simulink model "hvac_maborrelli_singapur_nzones_TCH2"  (R2021a)
settings: Solver=ode45  StartTime=0.0  StopTime=Inf  FixedStep=2  RelTol=1e-3  EnableMultiTasking=on
values from neighbouring files (symbols this model uses):
  beta = 0.15    [main_td3_nzones.m]
  ci = ci'    [localResetFcn.m]    (also in localResetFcnT.m)
  CO2_max = 1200*1e-6    (= 0.0012)    [main_td3_nzones.m]
  high = 25    [main_td3_nzones.m]    (also in reward.m)
  low = -10    [isDone.m]    (also in main_td3_nzones.m = 22; reward.m = 22)
  params = params1    [main_td3_nzones.m]
  paramsnz =     [values4z_tch.mat]
  scale = limit_act_low + limit_act_h    [main_td3_nzones.m]
  Ts = delta*Tr+(1-delta)*Toa + DT + DTH    [dynamics_hvac_maborrelli_singapur_1zone_tch.m]    (also in main_td3_nzones.m = 60)
  Ts2 = 900    [main.m]    (also in main_td3_nzones.m = 600)
undefined symbols (not defined in the file or in its folder): id, rl
libraries: simulink x6, dspmathops x5, rllib x1
settings Model: Creator=User  LastModifiedBy=Richi
settings SolverCC: AlgebraicLoopSolver=TrustRegion
settings DataIOCC: LimitDataPoints=on  SaveFormat=Array  SignalLoggingSaveFormat=ModelDataLogs
settings OptimizationCC: LifeSpan=inf
settings DebuggingCC: SolverPrmCheckMsg=warning  MultiTaskDSMMsg=warning  MultiTaskCondExecSysMsg=none  MultiTaskRateTransMsg=warning  StrictBusMsg=ErrorOnBusTreatedAsVector  SFUnexpectedBacktrackingDiag=warning  SFNoUnconditionalDefaultTransitionDiag=warning  SFExecutionAtInitializationDiag=none  SFMachineParentedDataDiag=warning  ArithmeticOperatorsInVariantConditions=warning
settings HardwareCC: ProdBitPerPointer=32  ProdBitPerSizeT=32  ProdBitPerPtrDiffT=32  ProdLargestAtomicFloat=None  ProdIntDivRoundTo=Undefined  ProdEndianess=Unspecified  ProdWordSize=32  ProdHWDeviceType=32-bit Generic
settings ModelReferenceCC: PropagateSignalLabelsOutOfModel=off
settings SFSimCC: SimUseLocalCustomCode=off  CustomCodeUndefinedFunction=UseInterfaceOnly
settings RTWCC: RTWUseLocalCustomCode=off
settings CodeAppCC: StateflowObjectComments=on
settings GRTTargetCC: TargetLangStandard=C89/C90 (ANSI)
settings ConfigComp: CovMetricSettings=dw  CovSaveCumulativeToWorkspaceVar=on  CovSaveSingleToWorkspaceVar=on  CovExternalEMLEnable=off

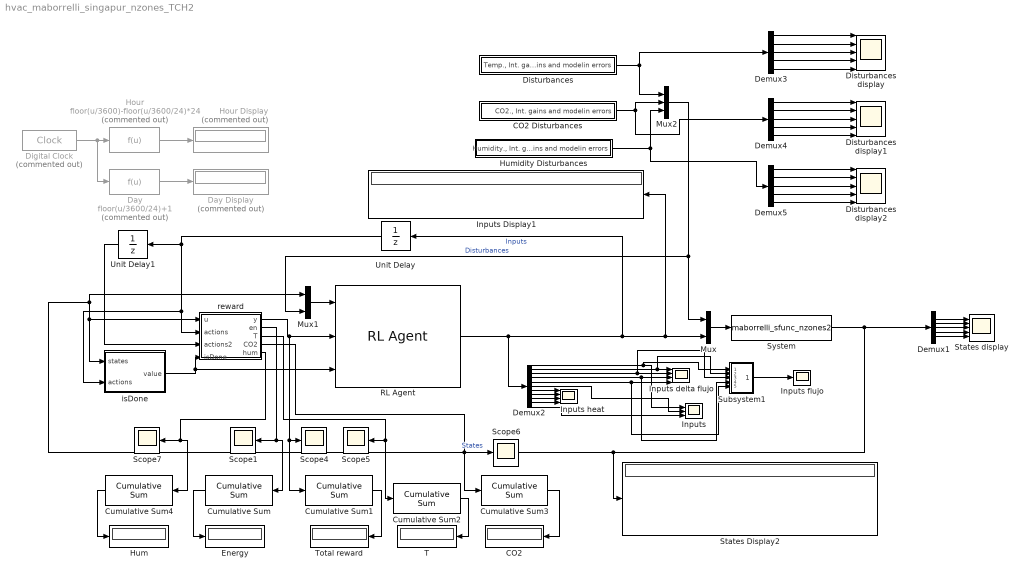
== system hvac_maborrelli_singapur_nzones_TCH2 ==
  CO2 : Display
  CO2 Disturbances : Subsystem  TreatAsAtomicUnit=on
  Cumulative Sum{,1..4} (5 alike) : dspmathops/Cumulative Sum  dim=Channels (running sum)  InputProcessing=Columns as channels (frame based)  reset_popup=None  roundingMode=Floor  overflowMode=off  outputDataTypeStr=Inherit: Same as accumulator  outputMin=[]  outputMax=[]  outputLastDataTypeStr=Inherit: Same as accumulator
  Day : Fcn  Commented=on  Expr=floor(u/3600/24)+1  SampleTime=1800
  Day Display : Display  Commented=on
  Demux{1,3..5} (4 alike) : Demux  Outputs=5
  Demux2 : Demux  Outputs=11
  Digital Clock : DigitalClock  Commented=on  SampleTime=60
  Disturbances : Subsystem  TreatAsAtomicUnit=on
  Disturbances display : Scope  NumInputPorts=5
  Disturbances display1 : Scope  NumInputPorts=5
  Disturbances display2 : Scope  NumInputPorts=5
  Energy : Display
  Hour : Fcn  Commented=on  Expr=floor(u/3600)-floor(u/3600/24)*24  SampleTime=1800
  Hour Display : Display  Commented=on
  Hum : Display
  Humidity Disturbances : Subsystem  TreatAsAtomicUnit=on
  "Inputs " : Scope  NumInputPorts=3
  Inputs Display1 : Display
  Inputs delta flujo : Scope  NumInputPorts=4
  Inputs flujo : Scope
  Inputs heat : Scope  NumInputPorts=4
  Mux : Mux  Inputs=2
  Mux1 : Mux  Inputs=2
  Mux2 : Mux  Inputs=3
  RL Agent : rllib/RL Agent  Agent=rl.util.PolicyInstance.get('hvac_maborrelli_singapur_nzones_with_MPC_v3_manualdist_3/RL Agent')  ExternalActionAsInput=off  ProvideCumRwd=off  TreatAsDirectFeedthrough=on
  Scope{1,4..7} (5 alike) : Scope
  States Display2 : Display
  States display : Scope  NumInputPorts=5
  Subsystem1 : Subsystem
  System : S-Function  FunctionName=maborrelli_sfunc_nzones2  Parameters=ci,paramsnz,Ts  SFunctionDeploymentMode=off  EnableBusSupport=off
  T : Display
  Total reward : Display
  Unit Delay : UnitDelay  SampleTime=Ts2  HasFrameUpgradeWarning=on
  Unit Delay1 : UnitDelay  SampleTime=Ts2  HasFrameUpgradeWarning=on
  isDone : MATLAB Function  TreatAsAtomicUnit=on
  reward : MATLAB Function  TreatAsAtomicUnit=on
  wires:
  Mux/1 -> System/1
  System/1 -> Demux1/1, States Display2/1, Mux1/1, isDone/1(states), reward/1(u)  "States"
  RL Agent/1 -> Unit Delay/1, Mux/2, Inputs Display1/1, Demux2/1  "Inputs"
  Hour/1 -> Hour Display/1
  Digital Clock/1 -> Day/1, Hour/1
  Day/1 -> Day Display/1
  Demux1/1 -> States display/1
  Demux1/2 -> States display/2
  Demux1/3 -> States display/3
  Demux1/4 -> States display/4
  isDone/1(value) -> reward/4(isDone), RL Agent/3
  Mux1/1 -> RL Agent/1
  Unit Delay/1 -> Unit Delay1/1, isDone/2(actions), reward/2(actions)
  Disturbances/1("Temp., Int. gains and modelin errors") -> Mux2/1, Demux3/1
  CO2 Disturbances/1("CO2., Int. gains and modelin errors") -> Mux2/2, Demux4/1
  Humidity Disturbances/1("Humidity., Int. gains and modelin errors") -> Demux5/1, Mux2/3
  Mux2/1 -> Mux1/2, Mux/1  "Disturbances"
  Demux3/1 -> Disturbances display/1
  Cumulative Sum4/1 -> Hum/1
  reward/4(CO2) -> Cumulative Sum3/1, Scope6/1
  Cumulative Sum/1 -> Energy/1
  Cumulative Sum2/1 -> T/1
  reward/5(hum) -> Cumulative Sum4/1, Scope7/1
  Cumulative Sum3/1 -> CO2/1
  reward/1(y) -> Cumulative Sum1/1, Scope4/1, RL Agent/2
  reward/3(T) -> Cumulative Sum2/1, Scope5/1
  Cumulative Sum1/1 -> Total reward/1
  reward/2(en) -> Cumulative Sum/1, Scope1/1
  Demux3/2 -> Disturbances display/2
  Demux3/3 -> Disturbances display/3
  Demux3/4 -> Disturbances display/4
  Demux3/5 -> Disturbances display/5
  Demux1/5 -> States display/5
  Demux4/4 -> Disturbances display1/4
  Demux4/2 -> Disturbances display1/2
  Demux4/3 -> Disturbances display1/3
  Demux4/1 -> Disturbances display1/1
  Demux4/5 -> Disturbances display1/5
  Demux5/4 -> Disturbances display2/4
  Demux5/2 -> Disturbances display2/2
  Demux5/3 -> Disturbances display2/3
  Demux5/1 -> Disturbances display2/1
  Demux5/5 -> Disturbances display2/5
  Unit Delay1/1 -> reward/3(actions2)
  Demux2/2 -> Subsystem1/2(In2), Inputs delta flujo/1
  Demux2/3 -> Inputs delta flujo/2, Subsystem1/3(In3)
  Demux2/4 -> Inputs delta flujo/3, Subsystem1/4(In4)
  Demux2/5 -> Inputs delta flujo/4, Subsystem1/5(In5)
  Demux2/1 -> Subsystem1/1(In1), "Inputs "/1
  Demux2/6 -> "Inputs "/2
  Demux2/11 -> "Inputs "/3
  Demux2/7 -> Inputs heat/1
  Demux2/8 -> Inputs heat/2
  Demux2/10 -> Inputs heat/4
  Demux2/9 -> Inputs heat/3
  Subsystem1/1(Out1) -> Inputs flujo/1

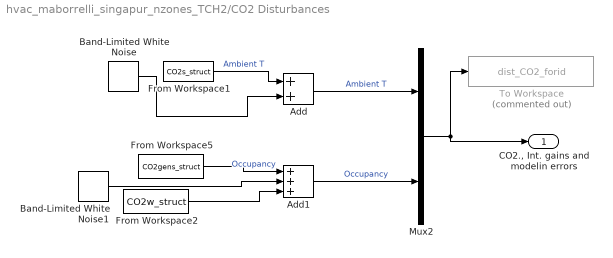
== system hvac_maborrelli_singapur_nzones_TCH2/CO2 Disturbances ==
  Add : Sum
  Add1 : Sum  Inputs=+++
  Band-Limited White Noise : simulink/Sources/Band-Limited White Noise  Cov=0  Ts=Ts  seed=[23341]
  Band-Limited White Noise1 : simulink/Sources/Band-Limited White Noise  Cov=0  Ts=Ts  seed=[23341]
  From Workspace1 : FromWorkspace  VariableName=CO2s_struct  OutDataTypeStr=double  SampleTime=Ts  ZeroCross=off
  From Workspace2 : FromWorkspace  VariableName=CO2w_struct  OutDataTypeStr=double  SampleTime=Ts  ZeroCross=off
  From Workspace5 : FromWorkspace  VariableName=CO2gens_struct  OutDataTypeStr=double  SampleTime=Ts  ZeroCross=off
  Mux2 : Mux  Inputs=2
  To Workspace : ToWorkspace  Commented=on  VariableName=dist_CO2_forid  SaveFormat=Timeseries  SampleTime=id.Delta
  "CO2., Int. gains and modelin errors" : Outport
  wires:
  From Workspace1/1 -> Add/1  "Ambient T"
  Band-Limited White Noise/1 -> Add/2
  Add/1 -> Mux2/1  "Ambient T"
  From Workspace5/1 -> Add1/1  "Occupancy"
  Band-Limited White Noise1/1 -> Add1/2
  From Workspace2/1 -> Add1/3
  Mux2/1 -> "CO2., Int. gains and modelin errors"/1, To Workspace/1
  Add1/1 -> Mux2/2  "Occupancy"

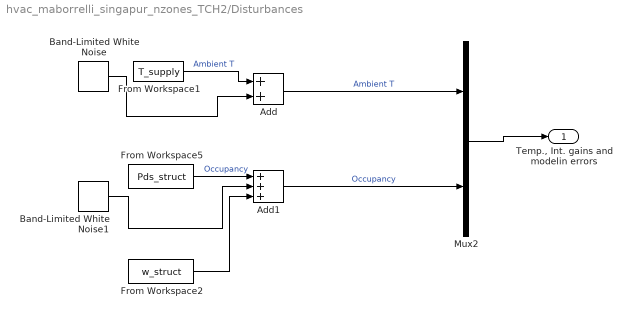
== system hvac_maborrelli_singapur_nzones_TCH2/Disturbances ==
  Add : Sum
  Add1 : Sum  Inputs=+++
  Band-Limited White Noise : simulink/Sources/Band-Limited White Noise  Cov=0  Ts=Ts2  seed=[23341]
  Band-Limited White Noise1 : simulink/Sources/Band-Limited White Noise  Cov=0  Ts=Ts2  seed=[23341]
  From Workspace1 : FromWorkspace  VariableName=T_supply  OutDataTypeStr=double  SampleTime=Ts  ZeroCross=off
  From Workspace2 : FromWorkspace  VariableName=w_struct  OutDataTypeStr=double  SampleTime=Ts  ZeroCross=off
  From Workspace5 : FromWorkspace  VariableName=Pds_struct  OutDataTypeStr=double  SampleTime=Ts  ZeroCross=off
  Mux2 : Mux  Inputs=2
  "Temp., Int. gains and modelin errors" : Outport
  wires:
  Add1/1 -> Mux2/2  "Occupancy"
  From Workspace1/1 -> Add/1  "Ambient T"
  Band-Limited White Noise/1 -> Add/2
  Add/1 -> Mux2/1  "Ambient T"
  From Workspace5/1 -> Add1/1  "Occupancy"
  Band-Limited White Noise1/1 -> Add1/2
  From Workspace2/1 -> Add1/3
  Mux2/1 -> "Temp., Int. gains and modelin errors"/1

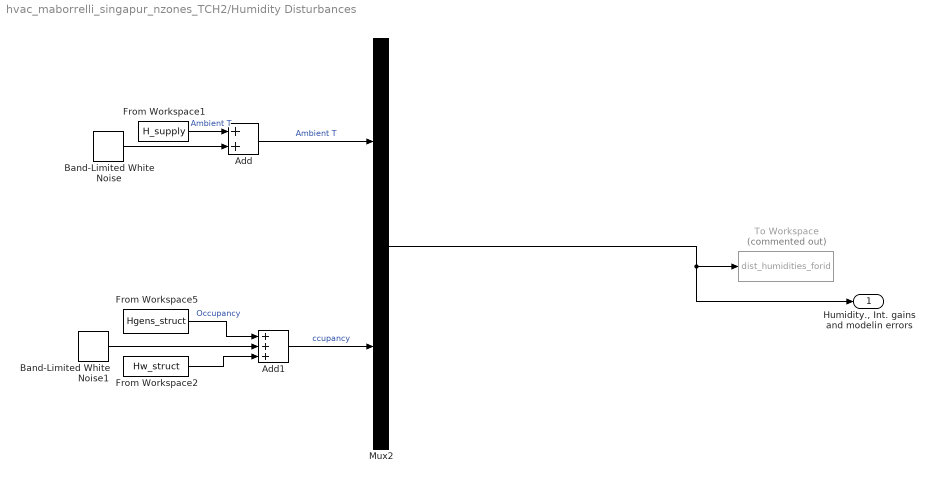
== system hvac_maborrelli_singapur_nzones_TCH2/Humidity Disturbances ==
  Add : Sum
  Add1 : Sum  Inputs=+++
  Band-Limited White Noise : simulink/Sources/Band-Limited White Noise  Cov=0  Ts=Ts  seed=[23341]
  Band-Limited White Noise1 : simulink/Sources/Band-Limited White Noise  Cov=0  Ts=Ts  seed=[23341]
  From Workspace1 : FromWorkspace  VariableName=H_supply  OutDataTypeStr=double  SampleTime=Ts  ZeroCross=off
  From Workspace2 : FromWorkspace  VariableName=Hw_struct  OutDataTypeStr=double  SampleTime=Ts  ZeroCross=off
  From Workspace5 : FromWorkspace  VariableName=Hgens_struct  OutDataTypeStr=double  SampleTime=Ts  ZeroCross=off
  Mux2 : Mux  Inputs=2
  To Workspace : ToWorkspace  Commented=on  VariableName=dist_humidities_forid  SaveFormat=Timeseries  SampleTime=id.Delta
  "Humidity., Int. gains and modelin errors" : Outport
  wires:
  From Workspace1/1 -> Add/1  "Ambient T"
  Band-Limited White Noise/1 -> Add/2
  Add/1 -> Mux2/1  "Ambient T"
  From Workspace5/1 -> Add1/1  "Occupancy"
  Band-Limited White Noise1/1 -> Add1/2
  From Workspace2/1 -> Add1/3
  Mux2/1 -> "Humidity., Int. gains and modelin errors"/1, To Workspace/1
  Add1/1 -> Mux2/2  "ccupancy"

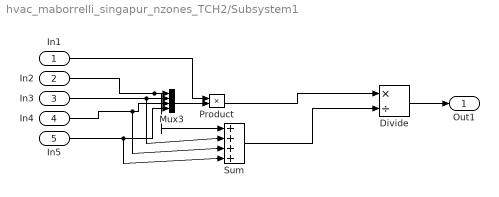
== system hvac_maborrelli_singapur_nzones_TCH2/Subsystem1 ==
  In1 : Inport
  In2 : Inport  Port=2
  In3 : Inport  Port=3
  In4 : Inport  Port=4
  In5 : Inport  Port=5
  Divide : Product  Inputs=*/
  Mux3 : Mux
  Product : Product
  Sum : Sum  Inputs=|++++
  Out1 : Outport
  wires:
  In5/1 -> Sum/4, Mux3/4
  In2/1 -> Sum/1, Mux3/1
  In4/1 -> Sum/3, Mux3/3
  In3/1 -> Sum/2, Mux3/2
  Divide/1 -> Out1/1
  In1/1 -> Product/1
  Mux3/1 -> Product/2
  Product/1 -> Divide/1
  Sum/1 -> Divide/2

== matlab function hvac_maborrelli_singapur_nzones_TCH2/isDone ==
  data: states input; value output; actions input
function value = isDone(states, actions)
 low = -0;
 max = 50;
 value = 0; 
 %disp(length(block.InputPort(1).Data))
 for i=1:length(states)
     if sum(actions(2:5)) > 5
         value = 1;
         break
     end
     %disp(i)
     if i <=4
        aux = states(i);
        if (aux < low || aux > max) 
            %disp(abs(aux - low))
            value = 1;
            break
        end
     elseif i>=9 && i<=12
        if states(i)>(3200*1e-6)
            value = 1;
            break
        end
     end
 end

== matlab function hvac_maborrelli_singapur_nzones_TCH2/reward ==
  data: u input; y output; actions input; actions2 input; isDone input; en output; T output; CO2 output; hum output; low parameter; high parameter; beta parameter; params parameter; CO2_max parameter; scale parameter
function [y, en, T,  CO2, hum] = reward(u ,  actions, actions2 , isDone, low, high, beta, params, CO2_max, scale)
 reward = 0;
 cp = params.cp;
 eta = params.eta;
 kf = params.kf;
 eta_h = params.eta_h;
 nz = 4;
 ms = actions(1:nz);
 Dt = actions(nz+1);
 Dth = actions(nz+2:2*nz+1);
 delta = actions(2*nz + 2);
 ms0 = actions2(1:nz);
 Dt0 = actions2(nz+1);
 Dth0 = actions2(nz+2:2*nz+1);
 delta0 = actions2(2*nz + 2);
 T_in = u(1:nz);
 CO2_in = u(2*nz+1:3*nz);
 hum_in = u(4*nz+1:5*nz);
 %Se inician las metricas
 CO2 = 0; hum = 0;T = 0;
 %Añadir energía:
 if sum(ms) > 5
     reward = -50;
 end
 %Energía utilizada por ventilador
 e = (kf*sum((ms).^2))/1000;
 %Energía por enfriar
 e = e + ((-cp/eta)*sum(ms)*(Dt))/1000;
 if abs(Dt0 - Dt) > 0.5*scale(nz+1)
     reward = reward - 10;
 end
 if abs(delta0 - delta) > 0.5*scale(2*nz + 2)
     reward = reward - 10;
 end
 for i=1:nz
     if abs(ms(i) - ms0(i)) > 0.5*scale(1)
        reward = reward - 10;
     end
     %Se aplica la penalización por energía al usar la calefacción
     if Dth(i) ~= 0
         e = e + ((cp/eta_h)*ms(i)*(Dth(i) - Dt))/1000;
     end
     %Se penaliza si hay calefacción pero no flujo de aire.
     if ms(i) == 0 && Dth(i)~=0
         reward = reward - 10;
     end
     %Se penaliza si hay enfriamiento pero no flujo de aire.
     if ms(i) == 0 && Dt~=0
         reward = reward - 0.5;
     end
     %Se penaliza romper las restricciones de temperatura.
     aux = T_in(i);
     if (aux < low || aux > high)
        T = T + 0.5*(min(abs(aux - low), abs(aux - high))+ (min( abs(aux - low), abs(aux - high)))^2);
        %reward = reward - T;
     %Entregar bonificación por estar en el estado
     else 
         reward = reward + 1;   
     end
     %Se penaliza romper las restricciones de concentración de CO2
     aux_co2 = CO2_in(i);
     if CO2_max < aux_co2
        CO2 = CO2 + abs(CO2_max - aux_co2)*30000;
        %reward = reward - CO2;
        if delta > 0.7
            reward = reward - 200;
        end
     end
     %Se penaliza romper las restricciones de humedad.
     Hum = hum_in(i);
     if (0.35 > Hum) || (Hum > 0.65)
         hum = hum + min(abs(Hum-0.35),abs(Hum-0.65));
         %reward = reward - hum;
     end
     
 %Se aplica el peso a la energía
 reward = reward - beta*e; 
 %Se aplica la penalización por estado
 reward = reward - T - CO2 - hum;
 en = e;
 end
 
 if isDone
     reward = -8000;
 end
y = reward;
